simulink model "HvCoorn"  (R2022b)
settings: configuration reference "Icar05FusaMdlCfg" (kept outside this file)
undefined symbols (not defined in the file): BMSActSt_ACChrg, BMSActSt_DCChrg, BMSActSt_disconnect, BMSActSt_offline, BMSActSt_online, BMSActSt_undefined, BMSMainNegRlySt_Clsd_SC, BMSMainNegRlySt_Open_SC, BMSMainNegRlySt_StuckInClsd_SC, BMSMainNegRlySt_StuckInOpen_SC, BMSMainPosRlySt_Clsd_SC, BMSMainPosRlySt_Open_SC, BMSMainPosRlySt_StuckInClsd_SC, BMSPrecRlySt_StuckInOpen_SC, BMSReqSt_ACChrg, BMSReqSt_DCChrg, BMSReqSt_emergencyOffline, BMSReqSt_offline, BMSReqSt_online, Chrg_stCycleBookMod_SC, Chrg_stSingleBookMod_SC, CmpgMod_stInactv_SC, DCDCActSt_buck, DCDCActSt_connected, DCDCActSt_disconnected, DCDCReqSt_buck, DCDCReqSt_standby, EngStrtStop_RefuModDft_SC, EPBActSt_Appld_SC, GearLvr_stDrvGearD_SC, GearLvr_stDrvGearN_SC, GearLvr_stDrvGearP_SC, GearLvr_stDrvGearR_SC, hpp_bACChargeLinkIni_C, hpp_bACChargeLinkOKIni_C, hpp_bAcChgEnaIni_C, hpp_bAcChgPauseIni_C, hpp_bAcLinkTempErrIni_C, hpp_bBattWarmReqIni_C, hpp_bHvilHwErrIni_C, hpp_bHvilStOkIni_C, hpp_bHvRelayClsActIni_C, hpp_bHvRelayOpnActIni_C, hpp_bHvRelayStuckIni_C, hpp_bParked4ChDchgIni_C, hpp_bRemLvBatMntnReqIni_C, hpp_bStartUpReqIni_C, hpp_stHvilCanIni_C, hpp_stWarmTimeCfgRespIni_C, HvCoorn_bAuthEnaSwt_C, HvCoorn_bAuthFailSpdLimOvrd_C, HvCoorn_bAuthFailSpdLimOvrdVal_C, HvCoorn_bAuthStrt_C, HvCoorn_bBMSUnexpdDcnctFailEna_C, HvCoorn_bBuck2RdyBypDCDCEna_C, HvCoorn_bDCChrgFctCfg_C, HvCoorn_bDcChrgWkupEnaChrgLink_C, HvCoorn_bDCDcnct4ACEna_C, HvCoorn_bDCNotBuck2ShtdwnEna_C, HvCoorn_bDrvrLevNotRdyEna_C ... (+295)
libraries: ITKLib x213, simulink x61
(part 1 of 12)
Description:
  | 本系统组件接收整车系统的上下高压需求，结合BMS/MCU/DCDC/OBC反馈的高压系统状态及整车车速/挡位等状态，管理协调高压上下电流程，并给BMS/MCU/DCDC等控制器发送相应的请求。
settings Model: Creator=shuliu1  LastModifiedBy=xuliu1
settings ConfigSetRef: SourceName=Icar05FusaMdlCfg  SourceLocation=Base Workspace

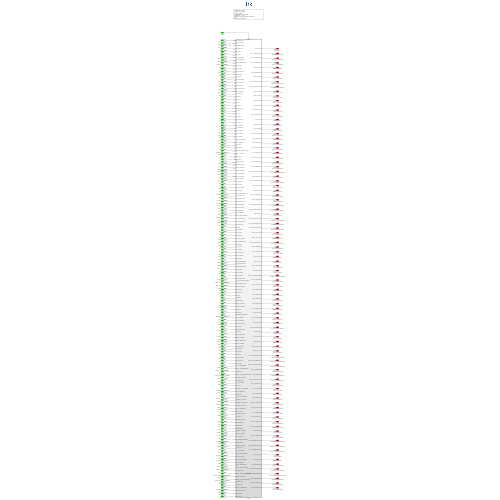
[thumbnail: Simulink's stored preview of the top-level diagram]
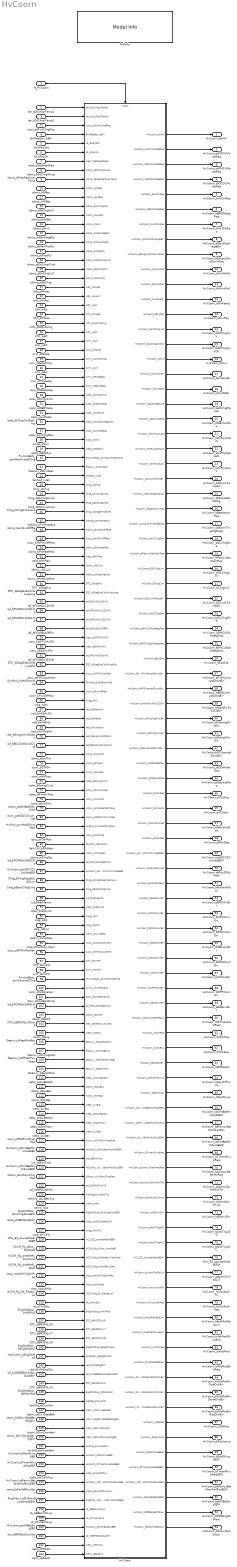
== system HvCoorn ==
  fc_HvCoorn : Inport  SampleTime=0.01  OutputFunctionCall=on
  ian_tDcChrgrTemp1 : Inport  Port=2  OutDataTypeStr=single
  ian_tDcChrgrTemp2 : Inport  Port=3  OutDataTypeStr=single
  BrkPedDev_bBrk : Inport  Port=4  OutDataTypeStr=boolean
  idi_bKeyStrt : Inport  Port=5  OutDataTypeStr=boolean
  idi_bKeyOn : Inport  Port=6  OutDataTypeStr=boolean
  icecc_bStalHeatReq : Inport  Port=7  OutDataTypeStr=boolean
  icbms_bDcChrgWkup : Inport  Port=8  OutDataTypeStr=boolean
  icbms_bPrecResOverTemp : Inport  Port=9  OutDataTypeStr=boolean
  icbms_iHVBat : Inport  Port=10  OutDataTypeStr=single
  icbms_uHVBat : Inport  Port=11  OutDataTypeStr=single
  icbms_bAcChrgFull : Inport  Port=12  OutDataTypeStr=boolean
  icbms_stHvBat : Inport  Port=13  OutDataTypeStr=uint8
  icbms_stHvil : Inport  Port=14  OutDataTypeStr=uint8
  icbms_stMainNegRly : Inport  Port=15  OutDataTypeStr=uint8
  icbms_stMainPosRly : Inport  Port=16  OutDataTypeStr=uint8
  icbms_stPrecRly : Inport  Port=17  OutDataTypeStr=uint8
  icbms_stDcChrgrCnct : Inport  Port=18  OutDataTypeStr=uint8
  icbms_bDcChrgFull : Inport  Port=19  OutDataTypeStr=boolean
  icbms_stDcChrg : Inport  Port=20  OutDataTypeStr=uint8
  icdc_stMode : Inport  Port=21  OutDataTypeStr=uint8
  icdc_uHvAct : Inport  Port=22  OutDataTypeStr=single
  icfm_nAct : Inport  Port=23  OutDataTypeStr=single
  icfm_stMode : Inport  Port=24  OutDataTypeStr=uint8
  icfm_stActvDchrg : Inport  Port=25  OutDataTypeStr=uint8
  icfm_uAct : Inport  Port=26  OutDataTypeStr=single
  icrm_nAct : Inport  Port=27  OutDataTypeStr=single
  icrm_stMode : Inport  Port=28  OutDataTypeStr=uint8
  icrm_stActvDchrg : Inport  Port=29  OutDataTypeStr=uint8
  icrm_uAct : Inport  Port=30  OutDataTypeStr=single
  icrm_stPlsHeatg : Inport  Port=31  OutDataTypeStr=uint8
  icrm_stStalHeatg : Inport  Port=32  OutDataTypeStr=uint8
  icobc_stChrgrCnct : Inport  Port=33  OutDataTypeStr=uint8
  icobc_stOBCMode : Inport  Port=34  OutDataTypeStr=uint8
  icobc_uHvDcAct : Inport  Port=35  OutDataTypeStr=single
  icobc_bChrgrCtrlSigCnct : Inport  Port=36  OutDataTypeStr=boolean
  icobc_pwrChrgMax : Inport  Port=37  OutDataTypeStr=single
  icobc_stHvil : Inport  Port=38  OutDataTypeStr=uint8
  icepb_stEpbSys : Inport  Port=39  OutDataTypeStr=uint8
  PwrLimBatt_pwrMaxHvesDChrg : Inport  Port=40  OutDataTypeStr=single
  GearLvr_stDrvGear : Inport  Port=41  OutDataTypeStr=uint8
  VehSpd_vVeh : Inport  Port=42  OutDataTypeStr=single
  Chrg_stChrg : Inport  Port=43  OutDataTypeStr=uint8
  Chrg_bACChrgCmpl : Inport  Port=44  OutDataTypeStr=boolean
  Chrg_bDCChrgCmpl : Inport  Port=45  OutDataTypeStr=boolean
  Chrg_bChrgErrForever : Inport  Port=46  OutDataTypeStr=boolean
  VehCfg_bFrntMotByp : Inport  Port=47  OutDataTypeStr=boolean
  icbms_bHvShutOffReq : Inport  Port=48  OutDataTypeStr=boolean
  iczcu_bHVPwrOffReq : Inport  Port=49  OutDataTypeStr=boolean
  icbms_bPlsHeatReq : Inport  Port=50  OutDataTypeStr=boolean
  icecc_bHVReq : Inport  Port=51  OutDataTypeStr=boolean
  icbms_uDCLnk : Inport  Port=52  OutDataTypeStr=single
  icbms_stPrechrgMod : Inport  Port=53  OutDataTypeStr=uint8
  DTC_bDiagEnaCdnWkupLong : Inport  Port=54  OutDataTypeStr=boolean
  ipf_bPCAN0x130Vld : Inport  Port=55  OutDataTypeStr=boolean
  ipf_bPCAN0x111S1Vld : Inport  Port=56  OutDataTypeStr=boolean
  ipf_bPCAN0x110S1Vld : Inport  Port=57  OutDataTypeStr=boolean
  ipf_bPCANBusOffErr : Inport  Port=58  OutDataTypeStr=boolean
  icecc_bWPTCHvilFlt : Inport  Port=59  OutDataTypeStr=boolean
  icecc_bEASHvilFlt : Inport  Port=60  OutDataTypeStr=boolean
  ipf_bPCAN0x353Vld : Inport  Port=61  OutDataTypeStr=boolean
  DTC_bDiagEnaCdnWkupSho : Inport  Port=62  OutDataTypeStr=boolean
  iczcu_stFMCUAuthent : Inport  Port=63  OutDataTypeStr=uint8
  DrvMod_bVehShowMod : Inport  Port=64  OutDataTypeStr=boolean
  icicm_bPwrOffReq : Inport  Port=65  OutDataTypeStr=boolean
  icisg_nAct : Inport  Port=66  OutDataTypeStr=single
  ved_bInhbHvOn : Inport  Port=67  OutDataTypeStr=boolean
  ved_bInhbRdy : Inport  Port=68  OutDataTypeStr=boolean
  ved_bHvShtdwn : Inport  Port=69  OutDataTypeStr=boolean
  ved_bEmgcyHvShtdwn : Inport  Port=70  OutDataTypeStr=boolean
  iczcu_stRmtChrgReq : Inport  Port=71  OutDataTypeStr=uint8
  ipf_bBD1CAN0x41CVld : Inport  Port=72  OutDataTypeStr=boolean
  icbms_stIsolTst : Inport  Port=73  OutDataTypeStr=uint8
  icicm_bOTAOn : Inport  Port=74  OutDataTypeStr=boolean
  icicm_stHVReq : Inport  Port=75  OutDataTypeStr=uint8
  icobc_bDchrgrCnct : Inport  Port=76  OutDataTypeStr=boolean
  ictcp_stRmtHvReq : Inport  Port=77  OutDataTypeStr=uint8
  icicm_stIvtrSwt : Inport  Port=78  OutDataTypeStr=uint8
  icbms_pctHVBatSOCDisp : Inport  Port=79  OutDataTypeStr=single
  icicm_pctSOCV2XLimSet : Inport  Port=80  OutDataTypeStr=single
  HvGrid_pwrMotDChrgMax : Inport  Port=81  OutDataTypeStr=single
  iczcu_stCarMod : Inport  Port=82  OutDataTypeStr=uint8
  ParkCtrl_bRPAActv : Inport  Port=83  OutDataTypeStr=boolean
  DTC_bDiagRst : Inport  Port=84  OutDataTypeStr=boolean
  icbms_stChrgSts : Inport  Port=85  OutDataTypeStr=uint8
  ipf_bPCAN0x343S2Vld : Inport  Port=86  OutDataTypeStr=boolean
  HvCoorn_pctSOCV2XLimSetEER : Inport  Port=87  OutDataTypeStr=single
  Chrg_bChrgStopBySOCLim : Inport  Port=88  OutDataTypeStr=boolean
  Chrg_bBookChrgCmpl : Inport  Port=89  OutDataTypeStr=boolean
  iud_bNetMaintn : Inport  Port=90  OutDataTypeStr=boolean
  icobc_bVehCnct : Inport  Port=91  OutDataTypeStr=boolean
  icisg_uAct : Inport  Port=92  OutDataTypeStr=single
  icisg_stMod : Inport  Port=93  OutDataTypeStr=uint8
  icdkm_stLrcpReq : Inport  Port=94  OutDataTypeStr=uint8
  ictcp_stLostComWarn : Inport  Port=95  OutDataTypeStr=uint8
  iczcu_stRMCUAuthent : Inport  Port=96  OutDataTypeStr=uint8
  icfm_bHvilFlt : Inport  Port=97  OutDataTypeStr=boolean
  icrm_bHvilFlt : Inport  Port=98  OutDataTypeStr=boolean
  PwrLimBatt_pwrContnsDChrg : Inport  Port=99  OutDataTypeStr=single
  icicm_stIvtrEnaSwt : Inport  Port=100  OutDataTypeStr=uint8
  ibsw_bCnctElecDvce : Inport  Port=101  OutDataTypeStr=boolean
  ipf_bPCAN0x340S1Vld : Inport  Port=102  OutDataTypeStr=boolean
  icbms_bIsolFlt : Inport  Port=103  OutDataTypeStr=boolean
  DTC_bBMSFltLvlOver5 : Inport  Port=104  OutDataTypeStr=boolean
  icems_stEng : Inport  Port=105  OutDataTypeStr=uint8
  GearLvr_bNapModActv : Inport  Port=106  OutDataTypeStr=boolean
  GearLvr_stCmpgMod : Inport  Port=107  OutDataTypeStr=uint8
  GearLvr_bOffVehPwrKeep : Inport  Port=108  OutDataTypeStr=boolean
  GearLvr_bSentilMod : Inport  Port=109  OutDataTypeStr=boolean
  icebs_pctLvBatSoh : Inport  Port=110  OutDataTypeStr=single
  icbms_tMaxBat : Inport  Port=111  OutDataTypeStr=single
  icbms_tMinBat : Inport  Port=112  OutDataTypeStr=single
  icebs_tLvBat : Inport  Port=113  OutDataTypeStr=single
  icebs_pctLvBatSoc : Inport  Port=114  OutDataTypeStr=single
  icebs_stSocPrcsn : Inport  Port=115  OutDataTypeStr=uint8
  icebs_uLvBat : Inport  Port=116  OutDataTypeStr=single
  icicm_stOTAPwrMngtReq : Inport  Port=117  OutDataTypeStr=uint8
  HvCoorn_ctSmtBatMntnFailEER : Inport  Port=118  OutDataTypeStr=uint8
  iud_bEEIniFnsd : Inport  Port=119  OutDataTypeStr=boolean
  HvCoorn_ctSmtBatMntnSucsEER : Inport  Port=120  OutDataTypeStr=uint16
  iclbms_stLvRemChrgReq : Inport  Port=121  OutDataTypeStr=uint8
  ipf_bLBMSCANVld : Inport  Port=122  OutDataTypeStr=boolean
  VehCfg_stLvBattTyp : Inport  Port=123  OutDataTypeStr=uint8
  icems_nAct : Inport  Port=124  OutDataTypeStr=single
  EngStrtStop_bFuChrgActvEEW : Inport  Port=125  OutDataTypeStr=boolean
  icobc_stOBCModeV2In : Inport  Port=126  OutDataTypeStr=uint8
  icisg_bHvilFlt : Inport  Port=127  OutDataTypeStr=boolean
  VCU_E2_counterfaieldEER : Inport  Port=128  OutDataTypeStr=uint8
  VCCM_flg_Allow_Antitheft : Inport  Port=129  OutDataTypeStr=boolean
  VCCM_flg_Antitheft_Overtime : Inport  Port=130  OutDataTypeStr=boolean
  VCCM_flg_Antitheft_Start : Inport  Port=131  OutDataTypeStr=boolean
  ictcp_noAuthChlgOnReq : Inport  Port=132  OutDataTypeStr=uint8  PortDimensions=[1 8]
  ictcp_noAuthSts : Inport  Port=133  OutDataTypeStr=uint8  PortDimensions=[1 8]
  VCCM_flg_SK_Recep_ok : Inport  Port=134  OutDataTypeStr=boolean
  idi_uPwrSply : Inport  Port=135  OutDataTypeStr=single
  EngStrtStop_bHVPRdy : Inport  Port=136  OutDataTypeStr=boolean
  DTC_bBMSFltLvl6 : Inport  Port=137  OutDataTypeStr=boolean
  DTC_bBMSFltLvl7 : Inport  Port=138  OutDataTypeStr=boolean
  DTC_bBMSFltLvl8 : Inport  Port=139  OutDataTypeStr=boolean
  EngStrtStop_bEngStrtAllw : Inport  Port=140  OutDataTypeStr=boolean
  HybCoorn_bEngStrtFail : Inport  Port=141  OutDataTypeStr=boolean
  ved_bInhbEngStrt : Inport  Port=142  OutDataTypeStr=boolean
  ipf_bLIN9EBS0x34NodLostErr : Inport  Port=143  OutDataTypeStr=boolean
  DTC_bBMSFltLvl5 : Inport  Port=144  OutDataTypeStr=boolean
  EngStrtStop_stRefuMod : Inport  Port=145  OutDataTypeStr=uint8
  VehCfg_stCycCdn : Inport  Port=146  OutDataTypeStr=uint8
  icbcm_stDrvrSeatBelt : Inport  Port=147  OutDataTypeStr=uint8
  icbcm_bStDrvrSeatBeltSigErr : Inport  Port=148  OutDataTypeStr=boolean
  icbcm_bDrvrDoorAjar : Inport  Port=149  OutDataTypeStr=boolean
  icbcm_bDrvrDoorAjarSigErr : Inport  Port=150  OutDataTypeStr=boolean
  HvGrid_pwrLoadAct : Inport  Port=151  OutDataTypeStr=single
  HvCoorn_bSocWkupEER : Inport  Port=152  OutDataTypeStr=boolean
  HvCoorn_bTimerWkupReqEER : Inport  Port=153  OutDataTypeStr=boolean
  icobc_stV2LFltTyp : Inport  Port=154  OutDataTypeStr=uint8
  HvCoorn_stRemLvBatMntnFailRsnEER : Inport  Port=155  OutDataTypeStr=uint8
  icems_bFanAftRunActv : Inport  Port=156  OutDataTypeStr=boolean
  RngPrdn_volFuRmnByInstModEEW : Inport  Port=157  OutDataTypeStr=single
  idi_bEBSLinWkup : Inport  Port=158  OutDataTypeStr=boolean
  idi_bTimerWkup : Inport  Port=159  OutDataTypeStr=boolean
  HvCoorn_pctHVBatSocEER : Inport  Port=160  OutDataTypeStr=single
  idi_noBMSSocCounter : Inport  Port=161  OutDataTypeStr=uint8
  icecc_uPTCAct : Inport  Port=162  OutDataTypeStr=single
  icecc_uEASAct : Inport  Port=163  OutDataTypeStr=single
  HvCoorn : Subsystem
      settings: LibrarySourceBlock=HvCoorn_stMac/HvCoorn_stMac/Subsystem/Subsystem
  MdlInfo : simulink/Model-Wide Utilities/Model Info  Frame=on  DisplayStringWithTags=|  HorizontalTextAlignment=Left  LeftAlignmentValue=0.02
      | <ModelName>: HvCoorn
      | <Project>: Chery_ICAR05
      | <Creator>: Li Shuai
      | <CreatedDate>: 2022 08 02 16:50
      | <ModelVersion>: 1.2.3.2
      | <Description>: High Voltage system Coordination
      | %<LastModifiedBy>
      | %<LastModificationDate>
  HvCoorn_stHVP : Outport  OutDataTypeStr=uint8
  HvCoorn_stFMCUModeReq : Outport  Port=2  OutDataTypeStr=uint8
  HvCoorn_stRMCUModeReq : Outport  Port=3  OutDataTypeStr=uint8
  HvCoorn_stDCDCModeReq : Outport  Port=4  OutDataTypeStr=uint8
  HvCoorn_bHvOnReq : Outport  Port=5  OutDataTypeStr=boolean
  HvCoorn_stBMSModeReq : Outport  Port=6  OutDataTypeStr=uint8
  HvCoorn_bHvilClsReq : Outport  Port=7  OutDataTypeStr=boolean
  HvCoorn_bActvDischargeErr : Outport  Port=8  OutDataTypeStr=boolean
  HvCoorn_bEmgcyShutDownReq : Outport  Port=9  OutDataTypeStr=boolean
  HvCoorn_bHvOnFail : Outport  Port=10  OutDataTypeStr=boolean
  HvCoorn_bHvInitFail : Outport  Port=11  OutDataTypeStr=boolean
  HvCoorn_bHvReady : Outport  Port=12  OutDataTypeStr=boolean
  HvCoorn_bDrvRdy : Outport  Port=13  OutDataTypeStr=boolean
  HvCoorn_bACChrgLink : Outport  Port=14  OutDataTypeStr=boolean
  HvCoorn_bACChrgLinkOk : Outport  Port=15  OutDataTypeStr=boolean
  HvCoorn_stHvil : Outport  Port=16  OutDataTypeStr=uint8
  HvCoorn_bHvilHwErr : Outport  Port=17  OutDataTypeStr=boolean
  HvCoorn_bHvilStOk : Outport  Port=18  OutDataTypeStr=boolean
  HvCoorn_bACChrgPause : Outport  Port=19  OutDataTypeStr=boolean
  HvCoorn_bStartUpReq : Outport  Port=20  OutDataTypeStr=boolean
  HvCoorn_bHvRlyClsAct : Outport  Port=21  OutDataTypeStr=boolean
  HvCoorn_bHvRlyOpenAct : Outport  Port=22  OutDataTypeStr=boolean
  HvCoorn_bHvRlyStuck : Outport  Port=23  OutDataTypeStr=boolean
  HvCoorn_bACLinkTempErr : Outport  Port=24  OutDataTypeStr=boolean
  HvCoorn_bParked4ChDchg : Outport  Port=25  OutDataTypeStr=boolean
  HvCoorn_bBattWarmReq : Outport  Port=26  OutDataTypeStr=boolean
  HvCoorn_stWarmTimeCfgResp : Outport  Port=27  OutDataTypeStr=uint8
  HvCoorn_bACChrgEna : Outport  Port=28  OutDataTypeStr=boolean
  HvCoorn_bRemLvBatMntnReq : Outport  Port=29  OutDataTypeStr=boolean
  HvCoorn_bDCChrgLink : Outport  Port=30  OutDataTypeStr=boolean
  HvCoorn_bChrgLink : Outport  Port=31  OutDataTypeStr=boolean
  HvCoorn_bDCLinkTempErr : Outport  Port=32  OutDataTypeStr=boolean
  HvCoorn_bDCChrgEna : Outport  Port=33  OutDataTypeStr=boolean
  HvCoorn_bRMCUPlsHeatgReq : Outport  Port=34  OutDataTypeStr=boolean
  HvCoorn_bRMCUStalHeatgReq : Outport  Port=35  OutDataTypeStr=boolean
  HvCoorn_bEccEna : Outport  Port=36  OutDataTypeStr=boolean
  HvCoorn_bHvRlyUnexpdDcnctErr : Outport  Port=37  OutDataTypeStr=boolean
  HvCoorn_bBMSUnexpdDcnctErr : Outport  Port=38  OutDataTypeStr=boolean
  HvCoorn_bMainRlyFail2ClsErr : Outport  Port=39  OutDataTypeStr=boolean
  HvCoorn_bPrechrgOvtiErr : Outport  Port=40  OutDataTypeStr=boolean
  HvCoorn_bDchrgOvtiErr : Outport  Port=41  OutDataTypeStr=boolean
  HvCoorn_bDCUnexpdDcnctErr : Outport  Port=42  OutDataTypeStr=boolean
  HvCoorn_stISGModeReq : Outport  Port=43  OutDataTypeStr=uint8
  HvCoorn_stStartUpReq : Outport  Port=44  OutDataTypeStr=uint8  VectorParamsAs1DForOutWhenUnconnected=off
  HvCoorn_bV2LActv : Outport  Port=45  OutDataTypeStr=boolean
  HvCoorn_bV2LReq : Outport  Port=46  OutDataTypeStr=boolean  VectorParamsAs1DForOutWhenUnconnected=off
  HvCoorn_bAllwShutNet : Outport  Port=47  OutDataTypeStr=boolean  VectorParamsAs1DForOutWhenUnconnected=off
  HvCoorn_bAllwSlep : Outport  Port=48  OutDataTypeStr=boolean  VectorParamsAs1DForOutWhenUnconnected=off
  HvCoorn_pctSOCV2XLimSetEEW : Outport  Port=49  OutDataTypeStr=single  VectorParamsAs1DForOutWhenUnconnected=off
  HvCoorn_stRdy2RdyWait : Outport  Port=50  OutDataTypeStr=uint8  VectorParamsAs1DForOutWhenUnconnected=off
  HvCoorn_bAuthentPass : Outport  Port=51  OutDataTypeStr=boolean  VectorParamsAs1DForOutWhenUnconnected=off
  HvCoorn_bBMSHvilErr : Outport  Port=52  OutDataTypeStr=boolean  VectorParamsAs1DForOutWhenUnconnected=off
  HvCoorn_bFMCUHvilErr : Outport  Port=53  OutDataTypeStr=boolean  VectorParamsAs1DForOutWhenUnconnected=off
  HvCoorn_bRMCUHvilErr : Outport  Port=54  OutDataTypeStr=boolean  VectorParamsAs1DForOutWhenUnconnected=off
  HvCoorn_bOBCHvilErr : Outport  Port=55  OutDataTypeStr=boolean  VectorParamsAs1DForOutWhenUnconnected=off
  HvCoorn_bDCDCHvilErr : Outport  Port=56  OutDataTypeStr=boolean  VectorParamsAs1DForOutWhenUnconnected=off
  HvCoorn_bHWHvilErr : Outport  Port=57  OutDataTypeStr=boolean  VectorParamsAs1DForOutWhenUnconnected=off
  HvCoorn_bWPTCHvilErr : Outport  Port=58  OutDataTypeStr=boolean  VectorParamsAs1DForOutWhenUnconnected=off
  HvCoorn_bEASHvilErr : Outport  Port=59  OutDataTypeStr=boolean  VectorParamsAs1DForOutWhenUnconnected=off
  HvCoorn_bMCUAuthentPass : Outport  Port=60  OutDataTypeStr=boolean  VectorParamsAs1DForOutWhenUnconnected=off
  HvCoorn_bV2InReq : Outport  Port=61  OutDataTypeStr=boolean  VectorParamsAs1DForOutWhenUnconnected=off
  HvCoorn_bV2InEna : Outport  Port=62  OutDataTypeStr=boolean  VectorParamsAs1DForOutWhenUnconnected=off
  HvCoorn_bBMSIsoErr : Outport  Port=63  OutDataTypeStr=boolean  VectorParamsAs1DForOutWhenUnconnected=off
  HvCoorn_bKeyOnPwrUp : Outport  Port=64  OutDataTypeStr=boolean  VectorParamsAs1DForOutWhenUnconnected=off
  HvCoorn_bSocWkup : Outport  Port=65  OutDataTypeStr=boolean  VectorParamsAs1DForOutWhenUnconnected=off
  HvCoorn_ctSmtBatMntnFailEEW : Outport  Port=66  OutDataTypeStr=uint8  VectorParamsAs1DForOutWhenUnconnected=off
  HvCoorn_stRemLvBatMntnFailRsn : Outport  Port=67  OutDataTypeStr=uint8  VectorParamsAs1DForOutWhenUnconnected=off
  HvCoorn_ctSmtBatMntnSucsEEW : Outport  Port=68  OutDataTypeStr=uint16  VectorParamsAs1DForOutWhenUnconnected=off
  HvCoorn_bTimerWkupReq : Outport  Port=69  OutDataTypeStr=boolean  VectorParamsAs1DForOutWhenUnconnected=off
  HvCoorn_bLbmsLvBatMntnReq : Outport  Port=70  OutDataTypeStr=boolean  VectorParamsAs1DForOutWhenUnconnected=off
  HvCoorn_pctLbmsSocMntnThd : Outport  Port=71  OutDataTypeStr=single  VectorParamsAs1DForOutWhenUnconnected=off
  HvCoorn_bLbmsSocWkup : Outport  Port=72  OutDataTypeStr=boolean  VectorParamsAs1DForOutWhenUnconnected=off
  HvCoorn_bISGHvilErr : Outport  Port=73  OutDataTypeStr=boolean  VectorParamsAs1DForOutWhenUnconnected=off
  HvCoorn_bAntiTrig430 : Outport  Port=74  OutDataTypeStr=boolean  VectorParamsAs1DForOutWhenUnconnected=off
  HvCoorn_bAntiTrig42C : Outport  Port=75  OutDataTypeStr=boolean  VectorParamsAs1DForOutWhenUnconnected=off
  VCU_E2_counterfaieldEEW : Outport  Port=76  OutDataTypeStr=uint8  VectorParamsAs1DForOutWhenUnconnected=off
  HvCoorn_stAuthChkFailLvl : Outport  Port=77  OutDataTypeStr=uint8  VectorParamsAs1DForOutWhenUnconnected=off
  HvCoorn_noVcuAuthFb : Outport  Port=78  OutDataTypeStr=uint8  PortDimensions=[1 8]  VectorParamsAs1DForOutWhenUnconnected=off
  HvCoorn_noVcuAuthReq : Outport  Port=79  OutDataTypeStr=uint8  PortDimensions=[1 8]  VectorParamsAs1DForOutWhenUnconnected=off
  HvCoorn_bAuthFailSpdLim : Outport  Port=80  OutDataTypeStr=boolean  VectorParamsAs1DForOutWhenUnconnected=off
  HvCoorn_bVehNetWkupEna : Outport  Port=81  OutDataTypeStr=boolean  VectorParamsAs1DForOutWhenUnconnected=off
  HvCoorn_stVoltMod : Outport  Port=82  OutDataTypeStr=uint8  VectorParamsAs1DForOutWhenUnconnected=off
  HvCoorn_bVoltModStbReq : Outport  Port=83  OutDataTypeStr=boolean  VectorParamsAs1DForOutWhenUnconnected=off
  HvCoorn_bVoltModHvDisbOvtiErr : Outport  Port=84  OutDataTypeStr=boolean  VectorParamsAs1DForOutWhenUnconnected=off
  HvCoorn_bVoltModHvDcnctOvtiErr : Outport  Port=85  OutDataTypeStr=boolean  VectorParamsAs1DForOutWhenUnconnected=off
  HvCoorn_bVoltModHvReqOvtiErr : Outport  Port=86  OutDataTypeStr=boolean  VectorParamsAs1DForOutWhenUnconnected=off
  HvCoorn_uISGReq : Outport  Port=87  OutDataTypeStr=single  VectorParamsAs1DForOutWhenUnconnected=off
  HvCoorn_bRdyLamp : Outport  Port=88  OutDataTypeStr=boolean
  HvCoorn_bSocWkupEEW : Outport  Port=89  OutDataTypeStr=boolean  VectorParamsAs1DForOutWhenUnconnected=off
  HvCoorn_bTimerWkupReqEEW : Outport  Port=90  OutDataTypeStr=boolean  VectorParamsAs1DForOutWhenUnconnected=off
  HvCoorn_stRemLvBatMntnFailRsnEEW : Outport  Port=91  OutDataTypeStr=uint8  VectorParamsAs1DForOutWhenUnconnected=off
  HvCoorn_pctHVBatSocEEW : Outport  Port=92  OutDataTypeStr=single  VectorParamsAs1DForOutWhenUnconnected=off
  HvCoorn_bDft2EngStrtRaw : Outport  Port=93  OutDataTypeStr=boolean  VectorParamsAs1DForOutWhenUnconnected=off
  HvCoorn_bShowModSocLo : Outport  Port=94  OutDataTypeStr=boolean  VectorParamsAs1DForOutWhenUnconnected=off
  wires:
  icbms_stMainPosRly/1 -> HvCoorn/16(icbms_stMainPosRly)
  icbms_stHvil/1 -> HvCoorn/14(icbms_stHvil)
  icbms_bDcChrgFull/1 -> HvCoorn/19(icbms_bDcChrgFull)
  icbms_stDcChrgrCnct/1 -> HvCoorn/18(icbms_stDcChrgrCnct)
  icdc_stMode/1 -> HvCoorn/21(icdc_stMode)
  icbms_stPrecRly/1 -> HvCoorn/17(icbms_stPrecRly)
  icbms_stMainNegRly/1 -> HvCoorn/15(icbms_stMainNegRly)
  icbms_stDcChrg/1 -> HvCoorn/20(icbms_stDcChrg)
  icecc_bStalHeatReq/1 -> HvCoorn/7(icecc_bStalHeatReq)
  icbms_bAcChrgFull/1 -> HvCoorn/12(icbms_bAcChrgFull)
  icbms_bDcChrgWkup/1 -> HvCoorn/8(icbms_bDcChrgWkup)
  icbms_stHvBat/1 -> HvCoorn/13(icbms_stHvBat)
  icbms_uHVBat/1 -> HvCoorn/11(icbms_uHVBat)
  icbms_iHVBat/1 -> HvCoorn/10(icbms_iHVBat)
  idi_bKeyOn/1 -> HvCoorn/6(idi_bKeyOn)
  idi_bKeyStrt/1 -> HvCoorn/5(idi_bKeyStrt)
  VehCfg_bFrntMotByp/1 -> HvCoorn/47(VehCfg_bFrntMotByp)
  Chrg_bDCChrgCmpl/1 -> HvCoorn/45(Chrg_bDCChrgCmpl)
  Chrg_bChrgErrForever/1 -> HvCoorn/46(Chrg_bChrgErrForever)
  GearLvr_stDrvGear/1 -> HvCoorn/41(GearLvr_stDrvGear)
  icobc_stHvil/1 -> HvCoorn/38(icobc_stHvil)
  icobc_pwrChrgMax/1 -> HvCoorn/37(icobc_pwrChrgMax)
  icobc_bChrgrCtrlSigCnct/1 -> HvCoorn/36(icobc_bChrgrCtrlSigCnct)
  icobc_uHvDcAct/1 -> HvCoorn/35(icobc_uHvDcAct)
  icrm_stActvDchrg/1 -> HvCoorn/29(icrm_stActvDchrg)
  icobc_stOBCMode/1 -> HvCoorn/34(icobc_stOBCMode)
  icfm_stActvDchrg/1 -> HvCoorn/25(icfm_stActvDchrg)
  icfm_uAct/1 -> HvCoorn/26(icfm_uAct)
  icdc_uHvAct/1 -> HvCoorn/22(icdc_uHvAct)
  icfm_stMode/1 -> HvCoorn/24(icfm_stMode)
  icrm_nAct/1 -> HvCoorn/27(icrm_nAct)
  icfm_nAct/1 -> HvCoorn/23(icfm_nAct)
  iczcu_stRmtChrgReq/1 -> HvCoorn/3(iczcu_stRmtChrgReq)
  icepb_stEpbSys/1 -> HvCoorn/39(icepb_stEpbSys)
  icrm_stPlsHeatg/1 -> HvCoorn/31(icrm_stPlsHeatg)
  icbms_bPrecResOverTemp/1 -> HvCoorn/9(icbms_bPrecResOverTemp)
  BrkPedDev_bBrk/1 -> HvCoorn/4(BrkPedDev_bBrk)
  icrm_uAct/1 -> HvCoorn/30(icrm_uAct)
  icobc_stChrgrCnct/1 -> HvCoorn/33(icobc_stChrgrCnct)
  icrm_stStalHeatg/1 -> HvCoorn/32(icrm_stStalHeatg)
  ian_tDcChrgrTemp1/1 -> HvCoorn/1(ian_tDcChrgrTemp1)
  ian_tDcChrgrTemp2/1 -> HvCoorn/2(ian_tDcChrgrTemp2)
  Chrg_stChrg/1 -> HvCoorn/43(Chrg_stChrg)
  icrm_stMode/1 -> HvCoorn/28(icrm_stMode)
  PwrLimBatt_pwrMaxHvesDChrg/1 -> HvCoorn/40(PwrLimBatt_pwrMaxHvesDChrg)
  VehSpd_vVeh/1 -> HvCoorn/42(VehSpd_vVeh)
  Chrg_bACChrgCmpl/1 -> HvCoorn/44(Chrg_bACChrgCmpl)
  icbms_bHvShutOffReq/1 -> HvCoorn/48(icbms_bHvShutOffReq)
  iczcu_bHVPwrOffReq/1 -> HvCoorn/49(iczcu_bHVPwrOffReq)
  icbms_bPlsHeatReq/1 -> HvCoorn/50(icbms_bPlsHeatReq)
  icecc_bHVReq/1 -> HvCoorn/51(icecc_bHVReq)
  icbms_uDCLnk/1 -> HvCoorn/52(icbms_uDCLnk)
  icbms_stPrechrgMod/1 -> HvCoorn/53(icbms_stPrechrgMod)
  DTC_bDiagRst/1 -> HvCoorn/54(DTC_bDiagRst)
  fc_HvCoorn/1 -> HvCoorn/Trigger
  HvCoorn/1(HvCoorn_stHVP) -> HvCoorn_stHVP/1
  HvCoorn/2(HvCoorn_stFMCUModeReq) -> HvCoorn_stFMCUModeReq/1
  HvCoorn/3(HvCoorn_stRMCUModeReq) -> HvCoorn_stRMCUModeReq/1
  HvCoorn/4(HvCoorn_stDCDCModeReq) -> HvCoorn_stDCDCModeReq/1
  HvCoorn/5(HvCoorn_bHvOnReq) -> HvCoorn_bHvOnReq/1
  HvCoorn/6(HvCoorn_stBMSModeReq) -> HvCoorn_stBMSModeReq/1
  HvCoorn/7(HvCoorn_bHvilClsReq) -> HvCoorn_bHvilClsReq/1
  HvCoorn/8(HvCoorn_bActvDischargeErr) -> HvCoorn_bActvDischargeErr/1
  HvCoorn/9(HvCoorn_bEmgcyShutDownReq) -> HvCoorn_bEmgcyShutDownReq/1
  HvCoorn/10(HvCoorn_bHvOnFail) -> HvCoorn_bHvOnFail/1
  HvCoorn/11(HvCoorn_bHvInitFail) -> HvCoorn_bHvInitFail/1
  HvCoorn/12(HvCoorn_bHvReady) -> HvCoorn_bHvReady/1
  HvCoorn/13(HvCoorn_bDrvRdy) -> HvCoorn_bDrvRdy/1
  HvCoorn/14(HvCoorn_bACChrgLink) -> HvCoorn_bACChrgLink/1
  HvCoorn/15(HvCoorn_bACChrgLinkOk) -> HvCoorn_bACChrgLinkOk/1
  HvCoorn/16(HvCoorn_stHvil) -> HvCoorn_stHvil/1
  HvCoorn/17(HvCoorn_bHvilHwErr) -> HvCoorn_bHvilHwErr/1
  HvCoorn/18(HvCoorn_bHvilStOk) -> HvCoorn_bHvilStOk/1
  HvCoorn/19(HvCoorn_bACChrgPause) -> HvCoorn_bACChrgPause/1
  HvCoorn/20(HvCoorn_bStartUpReq) -> HvCoorn_bStartUpReq/1
  HvCoorn/21(HvCoorn_bHvRlyClsAct) -> HvCoorn_bHvRlyClsAct/1
  HvCoorn/22(HvCoorn_bHvRlyOpenAct) -> HvCoorn_bHvRlyOpenAct/1
  HvCoorn/23(HvCoorn_bHvRlyStuck) -> HvCoorn_bHvRlyStuck/1
  HvCoorn/24(HvCoorn_bACLinkTempErr) -> HvCoorn_bACLinkTempErr/1
  HvCoorn/25(HvCoorn_bParked4ChDchg) -> HvCoorn_bParked4ChDchg/1
  HvCoorn/26(HvCoorn_bBattWarmReq) -> HvCoorn_bBattWarmReq/1
  HvCoorn/27(HvCoorn_stWarmTimeCfgResp) -> HvCoorn_stWarmTimeCfgResp/1
  HvCoorn/28(HvCoorn_bACChrgEna) -> HvCoorn_bACChrgEna/1
  HvCoorn/29(HvCoorn_bRemLvBatMntnReq) -> HvCoorn_bRemLvBatMntnReq/1
  HvCoorn/30(HvCoorn_bDCChrgLink) -> HvCoorn_bDCChrgLink/1
  HvCoorn/31(HvCoorn_bChrgLink) -> HvCoorn_bChrgLink/1
  HvCoorn/32(HvCoorn_bDCLinkTempErr) -> HvCoorn_bDCLinkTempErr/1
  HvCoorn/33(HvCoorn_bDCChrgEna) -> HvCoorn_bDCChrgEna/1
  HvCoorn/34(HvCoorn_bRMCUPlsHeatgReq) -> HvCoorn_bRMCUPlsHeatgReq/1
  HvCoorn/35(HvCoorn_bRMCUStalHeatgReq) -> HvCoorn_bRMCUStalHeatgReq/1
  HvCoorn/36(HvCoorn_bEccEna) -> HvCoorn_bEccEna/1
  HvCoorn/37(HvCoorn_bHvRlyUnexpdDcnctErr) -> HvCoorn_bHvRlyUnexpdDcnctErr/1
  HvCoorn/38(HvCoorn_bBMSUnexpdDcnctErr) -> HvCoorn_bBMSUnexpdDcnctErr/1
  HvCoorn/39(HvCoorn_bMainRlyFail2ClsErr) -> HvCoorn_bMainRlyFail2ClsErr/1
  HvCoorn/40(HvCoorn_bPrechrgOvtiErr) -> HvCoorn_bPrechrgOvtiErr/1
  HvCoorn/41(HvCoorn_bDchrgOvtiErr) -> HvCoorn_bDchrgOvtiErr/1
  HvCoorn/42(HvCoorn_bDCUnexpdDcnctErr) -> HvCoorn_bDCUnexpdDcnctErr/1
  DTC_bDiagEnaCdnWkupLong/1 -> HvCoorn/55(DTC_bDiagEnaCdnWkupLong)
  ipf_bPCAN0x130Vld/1 -> HvCoorn/56(ipf_bPCAN0x130Vld)
  ipf_bPCAN0x111S1Vld/1 -> HvCoorn/57(ipf_bPCAN0x111S1Vld)
  ipf_bPCAN0x110S1Vld/1 -> HvCoorn/58(ipf_bPCAN0x110S1Vld)
  ipf_bPCANBusOffErr/1 -> HvCoorn/59(ipf_bPCANBusOffErr)
  icecc_bWPTCHvilFlt/1 -> HvCoorn/60(icecc_bWPTCHvilFlt)
  icecc_bEASHvilFlt/1 -> HvCoorn/61(icecc_bEASHvilFlt)
  ipf_bPCAN0x353Vld/1 -> HvCoorn/62(ipf_bPCAN0x353Vld)
  DTC_bDiagEnaCdnWkupSho/1 -> HvCoorn/63(DTC_bDiagEnaCdnWkupSho)
  iczcu_stFMCUAuthent/1 -> HvCoorn/64(iczcu_stFMCUAuthent)
  DrvMod_bVehShowMod/1 -> HvCoorn/65(DrvMod_bVehShowMod)
  icicm_bPwrOffReq/1 -> HvCoorn/66(icicm_bPwrOffReq)
  icisg_nAct/1 -> HvCoorn/67(icisg_nAct)
  HvCoorn/43(HvCoorn_stISGModeReq) -> HvCoorn_stISGModeReq/1
  ved_bInhbHvOn/1 -> HvCoorn/68(ved_bInhbHvOn)
  ved_bInhbRdy/1 -> HvCoorn/69(ved_bInhbRdy)
  ved_bHvShtdwn/1 -> HvCoorn/70(ved_bHvShtdwn)
  ved_bEmgcyHvShtdwn/1 -> HvCoorn/71(ved_bEmgcyHvShtdwn)
  ipf_bBD1CAN0x41CVld/1 -> HvCoorn/72(ipf_bBD1CAN0x41CVld)
  icbms_stIsolTst/1 -> HvCoorn/73(icbms_stIsolTst)
  icicm_bOTAOn/1 -> HvCoorn/74(icicm_bOTAOn)
  icicm_stHVReq/1 -> HvCoorn/75(icicm_stHVReq)
  icobc_bDchrgrCnct/1 -> HvCoorn/76(icobc_bDchrgrCnct)
  HvCoorn/44(HvCoorn_stStartUpReq) -> HvCoorn_stStartUpReq/1
  ictcp_stRmtHvReq/1 -> HvCoorn/77(ictcp_stRmtHvReq)
  icicm_stIvtrSwt/1 -> HvCoorn/78(icicm_stIvtrSwt)
  icbms_pctHVBatSOCDisp/1 -> HvCoorn/79(icbms_pctHVBatSOCDisp)
  icicm_pctSOCV2XLimSet/1 -> HvCoorn/80(icicm_pctSOCV2XLimSet)
  HvGrid_pwrMotDChrgMax/1 -> HvCoorn/81(HvGrid_pwrMotDChrgMax)
  HvCoorn/46(HvCoorn_bV2LActv) -> HvCoorn_bV2LActv/1
  HvCoorn/45(HvCoorn_bV2LReq) -> HvCoorn_bV2LReq/1
  HvCoorn/47(HvCoorn_bAllwShutNet) -> HvCoorn_bAllwShutNet/1
  HvCoorn/48(HvCoorn_bAllwSlep) -> HvCoorn_bAllwSlep/1
  iczcu_stCarMod/1 -> HvCoorn/82(iczcu_stCarMod)
  ParkCtrl_bRPAActv/1 -> HvCoorn/83(ParkCtrl_bRPAActv)
  icbms_stChrgSts/1 -> HvCoorn/84(icbms_stChrgSts)
  ipf_bPCAN0x343S2Vld/1 -> HvCoorn/85(ipf_bPCAN0x343S2Vld)
  HvCoorn_pctSOCV2XLimSetEER/1 -> HvCoorn/86(HvCoorn_pctSOCV2XLimSetEER)
  HvCoorn/49(HvCoorn_pctSOCV2XLimSetEEW) -> HvCoorn_pctSOCV2XLimSetEEW/1
  Chrg_bChrgStopBySOCLim/1 -> HvCoorn/87(Chrg_bChrgStopBySOCLim)
  Chrg_bBookChrgCmpl/1 -> HvCoorn/88(Chrg_bBookChrgCmpl)
  iud_bNetMaintn/1 -> HvCoorn/89(iud_bNetMaintn)
  icobc_bVehCnct/1 -> HvCoorn/90(icobc_bVehCnct)
  HvCoorn/50(HvCoorn_stRdy2RdyWait) -> HvCoorn_stRdy2RdyWait/1
  HvCoorn/51(HvCoorn_bAuthentPass) -> HvCoorn_bAuthentPass/1
  icisg_uAct/1 -> HvCoorn/91(icisg_uAct)
  icisg_stMod/1 -> HvCoorn/92(icisg_stMod)
  icdkm_stLrcpReq/1 -> HvCoorn/93(icdkm_stLrcpReq)
  ictcp_stLostComWarn/1 -> HvCoorn/94(ictcp_stLostComWarn)
  HvCoorn/52(HvCoorn_bBMSHvilErr) -> HvCoorn_bBMSHvilErr/1
  HvCoorn/53(HvCoorn_bFMCUHvilErr) -> HvCoorn_bFMCUHvilErr/1
  HvCoorn/54(HvCoorn_bRMCUHvilErr) -> HvCoorn_bRMCUHvilErr/1
  HvCoorn/55(HvCoorn_bOBCHvilErr) -> HvCoorn_bOBCHvilErr/1
  HvCoorn/56(HvCoorn_bDCDCHvilErr) -> HvCoorn_bDCDCHvilErr/1
  HvCoorn/57(HvCoorn_bHWHvilErr) -> HvCoorn_bHWHvilErr/1
  HvCoorn/58(HvCoorn_bWPTCHvilErr) -> HvCoorn_bWPTCHvilErr/1
  HvCoorn/59(HvCoorn_bEASHvilErr) -> HvCoorn_bEASHvilErr/1
  iczcu_stRMCUAuthent/1 -> HvCoorn/95(iczcu_stRMCUAuthent)
  icfm_bHvilFlt/1 -> HvCoorn/96(icfm_bHvilFlt)
  icrm_bHvilFlt/1 -> HvCoorn/97(icrm_bHvilFlt)
  HvCoorn/60(HvCoorn_bMCUAuthentPass) -> HvCoorn_bMCUAuthentPass/1
  PwrLimBatt_pwrContnsDChrg/1 -> HvCoorn/98(PwrLimBatt_pwrContnsDChrg)
  icicm_stIvtrEnaSwt/1 -> HvCoorn/99(icicm_stIvtrEnaSwt)
  ibsw_bCnctElecDvce/1 -> HvCoorn/100(ibsw_bCnctElecDvce)
  HvCoorn/61(HvCoorn_bV2InReq) -> HvCoorn_bV2InReq/1
  HvCoorn/62(HvCoorn_bV2InEna) -> HvCoorn_bV2InEna/1
  ipf_bPCAN0x340S1Vld/1 -> HvCoorn/101(ipf_bPCAN0x340S1Vld)
  icbms_bIsolFlt/1 -> HvCoorn/102(icbms_bIsolFlt)
  DTC_bBMSFltLvlOver5/1 -> HvCoorn/103(DTC_bBMSFltLvlOver5)
  HvCoorn/63(HvCoorn_bBMSIsoErr) -> HvCoorn_bBMSIsoErr/1
  icems_stEng/1 -> HvCoorn/104(icems_stEng)
  GearLvr_bNapModActv/1 -> HvCoorn/105(GearLvr_bNapModActv)
  GearLvr_stCmpgMod/1 -> HvCoorn/106(GearLvr_stCmpgMod)
  GearLvr_bOffVehPwrKeep/1 -> HvCoorn/107(GearLvr_bOffVehPwrKeep)
  GearLvr_bSentilMod/1 -> HvCoorn/108(GearLvr_bSentilMod)
  icebs_pctLvBatSoh/1 -> HvCoorn/109(icebs_pctLvBatSoh)
  icbms_tMaxBat/1 -> HvCoorn/110(icbms_tMaxBat)
  icbms_tMinBat/1 -> HvCoorn/111(icbms_tMinBat)
  icebs_tLvBat/1 -> HvCoorn/112(icebs_tLvBat)
  icebs_pctLvBatSoc/1 -> HvCoorn/113(icebs_pctLvBatSoc)
  icebs_stSocPrcsn/1 -> HvCoorn/114(icebs_stSocPrcsn)
  icebs_uLvBat/1 -> HvCoorn/115(icebs_uLvBat)
  icicm_stOTAPwrMngtReq/1 -> HvCoorn/116(icicm_stOTAPwrMngtReq)
  HvCoorn_ctSmtBatMntnFailEER/1 -> HvCoorn/117(HvCoorn_ctSmtBatMntnFailEER)
  iud_bEEIniFnsd/1 -> HvCoorn/118(iud_bEEIniFnsd)
  HvCoorn/64(HvCoorn_bKeyOnPwrUp) -> HvCoorn_bKeyOnPwrUp/1
  HvCoorn/65(HvCoorn_bSocWkup) -> HvCoorn_bSocWkup/1
  HvCoorn/66(HvCoorn_ctSmtBatMntnFailEEW) -> HvCoorn_ctSmtBatMntnFailEEW/1
  HvCoorn/67(HvCoorn_stRemLvBatMntnFailRsn) -> HvCoorn_stRemLvBatMntnFailRsn/1
  HvCoorn/68(HvCoorn_ctSmtBatMntnSucsEEW) -> HvCoorn_ctSmtBatMntnSucsEEW/1
  HvCoorn_ctSmtBatMntnSucsEER/1 -> HvCoorn/119(HvCoorn_ctSmtBatMntnSucsEER)
  HvCoorn/69(HvCoorn_bTimerWkupReq) -> HvCoorn_bTimerWkupReq/1
  iclbms_stLvRemChrgReq/1 -> HvCoorn/120(iclbms_stLvRemChrgReq)
  ipf_bLBMSCANVld/1 -> HvCoorn/121(ipf_bLBMSCANVld)
  VehCfg_stLvBattTyp/1 -> HvCoorn/122(VehCfg_stLvBattTyp)
  HvCoorn/70(HvCoorn_bLbmsLvBatMntnReq) -> HvCoorn_bLbmsLvBatMntnReq/1
  HvCoorn/71(HvCoorn_pctLbmsSocMntnThd) -> HvCoorn_pctLbmsSocMntnThd/1
  HvCoorn/72(HvCoorn_bLbmsSocWkup) -> HvCoorn_bLbmsSocWkup/1
  icems_nAct/1 -> HvCoorn/123(icems_nAct)
  EngStrtStop_bFuChrgActvEEW/1 -> HvCoorn/124(EngStrtStop_bFuChrgActvEEW)
  icobc_stOBCModeV2In/1 -> HvCoorn/125(icobc_stOBCModeV2In)
  icisg_bHvilFlt/1 -> HvCoorn/126(icisg_bHvilFlt)
  HvCoorn/73(HvCoorn_bISGHvilErr) -> HvCoorn_bISGHvilErr/1
  VCU_E2_counterfaieldEER/1 -> HvCoorn/127(VCU_E2_counterfaieldEER)
  VCCM_flg_Allow_Antitheft/1 -> HvCoorn/128(VCCM_flg_Allow_Antitheft)
  VCCM_flg_Antitheft_Overtime/1 -> HvCoorn/129(VCCM_flg_Antitheft_Overtime)
  VCCM_flg_Antitheft_Start/1 -> HvCoorn/130(VCCM_flg_Antitheft_Start)
  ictcp_noAuthChlgOnReq/1 -> HvCoorn/131(ictcp_noAuthChlgOnReq)
  ictcp_noAuthSts/1 -> HvCoorn/132(ictcp_noAuthSts)
  VCCM_flg_SK_Recep_ok/1 -> HvCoorn/133(VCCM_flg_SK_Recep_ok)
  HvCoorn/74(HvCoorn_bAntiTrig430) -> HvCoorn_bAntiTrig430/1
  HvCoorn/75(HvCoorn_bAntiTrig42C) -> HvCoorn_bAntiTrig42C/1
  HvCoorn/76(VCU_E2_counterfaieldEEW) -> VCU_E2_counterfaieldEEW/1
  HvCoorn/77(HvCoorn_stAuthChkFailLvl) -> HvCoorn_stAuthChkFailLvl/1
  HvCoorn/78(HvCoorn_noVcuAuthFb) -> HvCoorn_noVcuAuthFb/1
  HvCoorn/79(HvCoorn_noVcuAuthReq) -> HvCoorn_noVcuAuthReq/1
  HvCoorn/80(HvCoorn_bAuthFailSpdLim) -> HvCoorn_bAuthFailSpdLim/1
  idi_uPwrSply/1 -> HvCoorn/134(idi_uPwrSply)
  HvCoorn/81(HvCoorn_bVehNetWkupEna) -> HvCoorn_bVehNetWkupEna/1
  EngStrtStop_bHVPRdy/1 -> HvCoorn/135(EngStrtStop_bHVPRdy)
  DTC_bBMSFltLvl6/1 -> HvCoorn/136(DTC_bBMSFltLvl6)
  DTC_bBMSFltLvl7/1 -> HvCoorn/137(DTC_bBMSFltLvl7)
  DTC_bBMSFltLvl8/1 -> HvCoorn/138(DTC_bBMSFltLvl8)
  EngStrtStop_bEngStrtAllw/1 -> HvCoorn/139(EngStrtStop_bEngStrtAllw)
  HybCoorn_bEngStrtFail/1 -> HvCoorn/140(HybCoorn_bEngStrtFail)
  ved_bInhbEngStrt/1 -> HvCoorn/141(ved_bInhbEngStrt)
  HvCoorn/82(HvCoorn_stVoltMod) -> HvCoorn_stVoltMod/1
  HvCoorn/83(HvCoorn_bVoltModStbReq) -> HvCoorn_bVoltModStbReq/1
  HvCoorn/84(HvCoorn_bVoltModHvDisbOvtiErr) -> HvCoorn_bVoltModHvDisbOvtiErr/1
  HvCoorn/85(HvCoorn_bVoltModHvDcnctOvtiErr) -> HvCoorn_bVoltModHvDcnctOvtiErr/1
  HvCoorn/86(HvCoorn_bVoltModHvReqOvtiErr) -> HvCoorn_bVoltModHvReqOvtiErr/1
  HvCoorn/87(HvCoorn_uISGReq) -> HvCoorn_uISGReq/1
  ipf_bLIN9EBS0x34NodLostErr/1 -> HvCoorn/142(ipf_bLIN9EBS0x34NodLostErr)
  DTC_bBMSFltLvl5/1 -> HvCoorn/143(DTC_bBMSFltLvl5)
  EngStrtStop_stRefuMod/1 -> HvCoorn/144(EngStrtStop_stRefuMod)
  VehCfg_stCycCdn/1 -> HvCoorn/145(VehCfg_stCycCdn)
  icbcm_stDrvrSeatBelt/1 -> HvCoorn/146(icbcm_stDrvrSeatBelt)
  icbcm_bStDrvrSeatBeltSigErr/1 -> HvCoorn/147(icbcm_bStDrvrSeatBeltSigErr)
  icbcm_bDrvrDoorAjar/1 -> HvCoorn/148(icbcm_bDrvrDoorAjar)
  icbcm_bDrvrDoorAjarSigErr/1 -> HvCoorn/149(icbcm_bDrvrDoorAjarSigErr)
  HvCoorn/88(HvCoorn_bRdyLamp) -> HvCoorn_bRdyLamp/1
  HvGrid_pwrLoadAct/1 -> HvCoorn/150(HvGrid_pwrLoadAct)
  HvCoorn_bSocWkupEER/1 -> HvCoorn/151(HvCoorn_bSocWkupEER)
  HvCoorn_bTimerWkupReqEER/1 -> HvCoorn/152(HvCoorn_bTimerWkupReqEER)
  HvCoorn/89(HvCoorn_bSocWkupEEW) -> HvCoorn_bSocWkupEEW/1
  HvCoorn/90(HvCoorn_bTimerWkupReqEEW) -> HvCoorn_bTimerWkupReqEEW/1
  icobc_stV2LFltTyp/1 -> HvCoorn/153(icobc_stV2LFltTyp)
  HvCoorn_stRemLvBatMntnFailRsnEER/1 -> HvCoorn/154(HvCoorn_stRemLvBatMntnFailRsnEER)
  HvCoorn/91(HvCoorn_stRemLvBatMntnFailRsnEEW) -> HvCoorn_stRemLvBatMntnFailRsnEEW/1
  icems_bFanAftRunActv/1 -> HvCoorn/155(icems_bFanAftRunActv)
  RngPrdn_volFuRmnByInstModEEW/1 -> HvCoorn/156(RngPrdn_volFuRmnByInstModEEW)
  idi_bEBSLinWkup/1 -> HvCoorn/157(idi_bEBSLinWkup)
  idi_bTimerWkup/1 -> HvCoorn/158(idi_bTimerWkup)
  HvCoorn_pctHVBatSocEER/1 -> HvCoorn/159(HvCoorn_pctHVBatSocEER)
  idi_noBMSSocCounter/1 -> HvCoorn/160(idi_noBMSSocCounter)
  HvCoorn/92(HvCoorn_pctHVBatSocEEW) -> HvCoorn_pctHVBatSocEEW/1
  HvCoorn/93(HvCoorn_bDft2EngStrtRaw) -> HvCoorn_bDft2EngStrtRaw/1
  HvCoorn/94(HvCoorn_bShowModSocLo) -> HvCoorn_bShowModSocLo/1
  icecc_uPTCAct/1 -> HvCoorn/161(icecc_uPTCAct)
  icecc_uEASAct/1 -> HvCoorn/162(icecc_uEASAct)
